simulink model "Example1_5"  (R2012a)
settings: Solver=ode45  StartTime=0.0  StopTime=T  MaxStep=MaxStep  RelTol=RelTol
values from neighbouring files (symbols this model uses):
  J = 20    [initialization_ex1_5.m]
  rule = 1    [initialization_ex1_5.m]
  T = 15    [initialization_ex1_5.m]
  x0 = [0; 0; pi/4; 2]    [initialization_ex1_5.m]
libraries: simulink x3
settings Model: Creator=pablonanez  LastModifiedBy=pablonanez
settings DataIOCC: LimitDataPoints=on  SaveFormat=Array  SignalLoggingSaveFormat=ModelDataLogs  ReturnWorkspaceOutputs=off
settings OptimizationCC: ExpressionDepthLimit=2147483647  LifeSpan=inf  SimCompilerOptimization=Off
settings DebuggingCC: UnderspecifiedInitializationDetection=Classic  MergeDetectMultiDrivingBlocksExec=none  SolverPrmCheckMsg=warning  FcnCallInpInsideContextMsg=Enable All  StateNameClashWarn=warning  SFUnexpectedBacktrackingDiag=warning  SFNoUnconditionalDefaultTransitionDiag=warning
settings HardwareCC: ProdBitPerPointer=32  ProdLargestAtomicFloat=None  ProdIntDivRoundTo=Undefined  ProdEndianess=Unspecified  ProdWordSize=32  ProdHWDeviceType=32-bit Generic
settings ModelReferenceCC: PropagateSignalLabelsOutOfModel=off
settings SFSimCC: SimUseLocalCustomCode=off  SimParseCustomCode=off
settings RTWCC: RTWUseLocalCustomCode=off  RTWCompilerOptimization=Off
settings GRTTargetCC: CodeReplacementLibrary=C89/C90 (ANSI)  GeneratePreprocessorConditionals=Disable all  CombineOutputUpdateFcns=off  CPPClassGenCompliant=off  GRTInterface=on

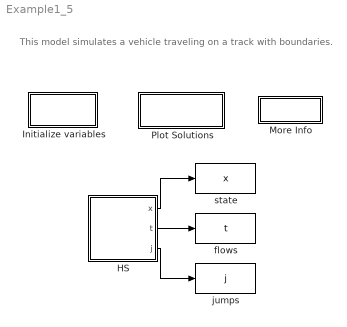
== system Example1_5 ==
  note: This model simulates a vehicle
      | traveling on a track with boundaries.
  HS : Subsystem  LoadFcn=set_param(gcb,'LinkStatus','none')
      settings: CopyFcn=|
      | set_param(gcb,'LinkStatus','none')
      | set_param(gcs, 'MaxStep', 'MaxStep', 'RelTol', 'RelTol')
      mask Display:
      | image(imread('Hcal.jpg'))
      | %plot([5 20 20 5 5],[5 5 20 20 5])
      | %text(8,13,'HyEq_mdl')
      | port_label('output', 1, 'x')
      | port_label('output', 2, 't')
      | port_label('output', 3, 'j')
  Initialize variables : Subsystem  Priority=-10
      settings: OpenFcn=initialization_ex1_5
      mask Display: disp('Double Click\n to Initialize')
  More Info : Subsystem
      settings: OpenFcn=web( 'Example_1_5.html')
      mask Display: disp('More Info')
  Plot Solutions : Subsystem
      settings: OpenFcn=postprocessing_ex1_5
      mask Display: disp('Double Click to\n Plot Solutions')
  flows : ToWorkspace  VariableName=t  SampleTime=-1
  jumps : ToWorkspace  VariableName=j  SampleTime=-1
  state : ToWorkspace  VariableName=x  SampleTime=-1
  wires:
  HS/2(t) -> flows/1
  HS/1(x) -> state/1
  HS/3(j) -> jumps/1

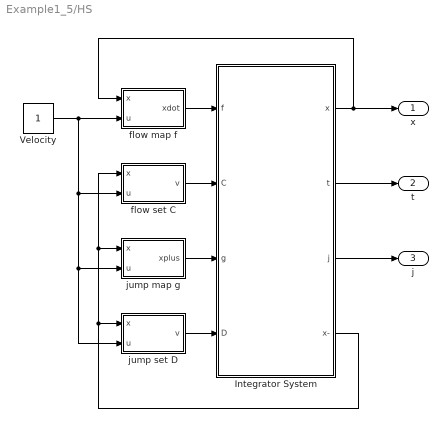
== system Example1_5/HS ==
  Integrator System : Subsystem  Priority=2  mask(Hybrid Integrator){T=T, J=J, x0=x0}
      mask prompts: T "Flow Horizon"; J "Jump Horizon"; x0 "Initial Condition"
      mask help:
      | This block integrates the state of the hybrid system defined by the flow map f (first input), the flow set C (second input), the jump map g (third input) and the jump set D (fourth input).
      | Starting from the initial condition x0 (last mask parameter), the system's state x evolves continuously within the set C, according to f(x,u), but is also subject to jumps within D, according to g(x,u).
      | The block also stops the simulation when the time t is greater than the flow horizon T (first mask parameter), or when the number of jumps j is greater than the jump horizon J (second mask parameter).
      | The outputs of the blocks are respectively x(t), t, j, x(t-).
      mask Help:
      | This block integrates the state of the hybrid system defined by the flow map f (first input), the flow set C (second input), the jump map g (third input) and the jump set D (fourth input).
      | <br>
      | Starting from the initial condition x0 (last mask parameter), the system's state x evolves continuously within the set C, according to f(x,u), but is also subject to jumps within D, according to g(x,u).
      | <br>
      | The block also stops the simulation when the time t is greater than the flow horizon T (first mask parameter), or when the number of jumps j is greater than the jump horizon J (second mask parameter).
      | <br>
      | The outputs of the blocks are respectively x(t), t, j, x(t-).
      | <br>
      | You can right click on the block and "Look under mask" to see what's inside the block.
      | Finally, refer to the manual (HybridSimulator_vXX.pdf) for more detailed information on how this hybrid simulator works.
  Velocity : Constant
  flow map f : MATLAB Function  TreatAsAtomicUnit=on
      settings: PermitHierarchicalResolution=ParametersOnly
  flow set C : MATLAB Function  TreatAsAtomicUnit=on
      settings: PermitHierarchicalResolution=ParametersOnly
  jump map g : MATLAB Function  Priority=2  TreatAsAtomicUnit=on
      settings: PermitHierarchicalResolution=ParametersOnly
  jump set D : MATLAB Function  TreatAsAtomicUnit=on
      settings: PermitHierarchicalResolution=ParametersOnly
  x : Outport
  t : Outport  Port=2
  j : Outport  Port=3
  wires:
  flow map f/1(xdot) -> Integrator System/1(f)
  Integrator System/4(x-) -> jump map g/1(x), flow set C/1(x), jump set D/1(x)
  Integrator System/1(x) -> flow map f/1(x), x/1
  flow set C/1(v) -> Integrator System/2(C)
  Integrator System/2(t) -> t/1
  Integrator System/3(j) -> j/1
  Velocity/1 -> flow map f/2(u), flow set C/2(u), jump map g/2(u), jump set D/2(u)
  jump set D/1(v) -> Integrator System/4(D)
  jump map g/1(xplus) -> Integrator System/3(g)

== system Example1_5/Initialize variables ==

== system Example1_5/More Info ==

== system Example1_5/Plot Solutions ==

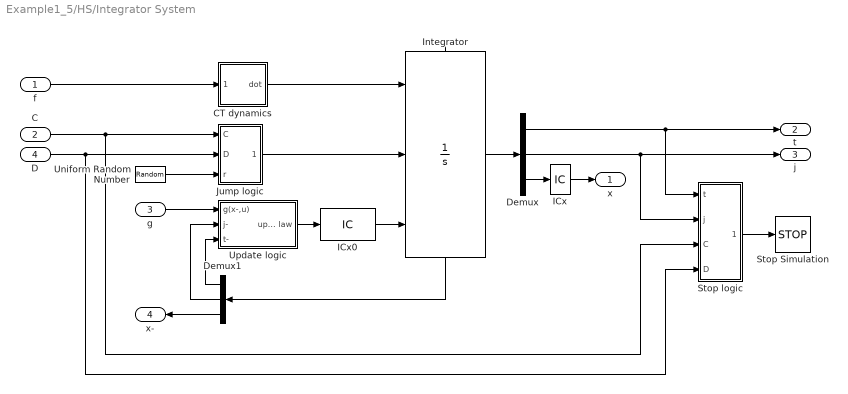
== system Example1_5/HS/Integrator System ==
  f : Inport
  C : Inport  Port=2
  g : Inport  Port=3
  D : Inport  Port=4
  CT dynamics : Subsystem
  Demux : Demux  Outputs=[1 1 -1]
  Demux1 : Demux  Outputs=[1 1 -1]
  ICx : InitialCondition  Value=x0
  ICx0 : InitialCondition  Value=[0; 0; x0(:)]
  Integrator : Integrator  ExternalReset=level hold  InitialConditionSource=external  ShowStatePort=on  ZeroCross=off
  Jump logic : Subsystem
  Stop Simulation : Stop
  Stop logic : Subsystem
  Uniform Random Number : UniformRandomNumber  Minimum=0  Seed=abs(floor(100*rand))  SampleTime=0
  Update logic : Subsystem
  x : Outport
  t : Outport  Port=2
  j : Outport  Port=3
  x- : Outport  Port=4
  wires:
  Demux1/2 -> Update logic/2(j-)
  Demux1/1 -> Update logic/3(t-)
  g/1 -> Update logic/1(g(x-,u))
  Uniform Random Number/1 -> Jump logic/3(r)
  Jump logic/1(jump) -> Integrator/2
  Demux1/3 -> x-/1
  f/1 -> CT dynamics/1(f(x,u))
  D/1 -> Jump logic/2(D), Stop logic/4(D)
  C/1 -> Jump logic/1(C), Stop logic/3(C)
  Integrator/1 -> Demux/1
  Stop logic/1(stop) -> Stop Simulation/1
  CT dynamics/1(dot) -> Integrator/1
  Update logic/1(update law) -> ICx0/1
  Demux/1 -> Stop logic/1(t), t/1
  Demux/2 -> Stop logic/2(j), j/1
  Integrator/State -> Demux1/1
  Demux/3 -> ICx/1
  ICx/1 -> x/1
  ICx0/1 -> Integrator/3

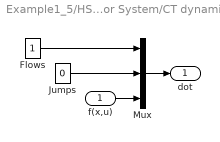
== system Example1_5/HS/Integrator System/CT dynamics ==
  f(x,u) : Inport
  Flows : Constant
  Jumps : Constant  Value=0
  Mux : Mux  Inputs=[1 1 -1]
  dot : Outport
  wires:
  f(x,u)/1 -> Mux/3
  Mux/1 -> dot/1
  Flows/1 -> Mux/1
  Jumps/1 -> Mux/2

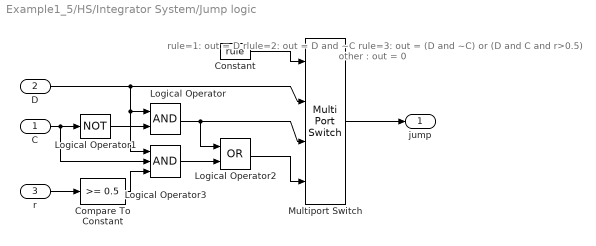
== system Example1_5/HS/Integrator System/Jump logic ==
  note: rule=1:  out = D
      | rlule=2: out = D and ~C
      | rule=3:  out = (D and ~C)  or (D and C and r>0.5)
      | other :  out = 0
  C : Inport
  D : Inport  Port=2
  r : Inport  Port=3
  Compare To Constant : simulink/Logic and Bit Operations/Compare To Constant  relop=>=  const=0.5  OutDataTypeStr=uint8
  Constant : Constant  Value=rule
  Logical Operator : Logic  AllPortsSameDT=off  OutDataTypeStr=boolean
  Logical Operator1 : Logic  Operator=NOT  Inputs=1  AllPortsSameDT=off  OutDataTypeStr=boolean
  Logical Operator2 : Logic  Operator=OR  AllPortsSameDT=off  OutDataTypeStr=boolean
  Logical Operator3 : Logic  Inputs=3  AllPortsSameDT=off  OutDataTypeStr=boolean
  Multiport Switch : MultiPortSwitch
  jump : Outport
  wires:
  Logical Operator3/1 -> Logical Operator2/2
  Compare To Constant/1 -> Logical Operator3/3
  Multiport Switch/1 -> jump/1
  Logical Operator2/1 -> Multiport Switch/4
  Logical Operator/1 -> Logical Operator2/1, Multiport Switch/3
  Logical Operator1/1 -> Logical Operator/2
  C/1 -> Logical Operator1/1, Logical Operator3/2
  r/1 -> Compare To Constant/1
  D/1 -> Multiport Switch/2, Logical Operator/1, Logical Operator3/1
  Constant/1 -> Multiport Switch/1

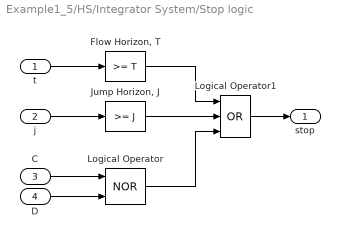
== system Example1_5/HS/Integrator System/Stop logic ==
  t : Inport
  j : Inport  Port=2
  C : Inport  Port=3
  D : Inport  Port=4
  "Flow Horizon, T" : simulink/Logic and Bit Operations/Compare To Constant  relop=>=  const=T  OutDataTypeStr=uint8  ZeroCross=off
  "Jump Horizon, J" : simulink/Logic and Bit Operations/Compare To Constant  relop=>=  const=J  OutDataTypeStr=uint8  ZeroCross=off
  Logical Operator : Logic  Operator=NOR  AllPortsSameDT=off  OutDataTypeStr=boolean
  Logical Operator1 : Logic  Operator=OR  Inputs=3  AllPortsSameDT=off  OutDataTypeStr=boolean
  stop : Outport
  wires:
  Logical Operator1/1 -> stop/1
  C/1 -> Logical Operator/1
  j/1 -> "Jump Horizon, J"/1
  t/1 -> "Flow Horizon, T"/1
  D/1 -> Logical Operator/2
  Logical Operator/1 -> Logical Operator1/3
  "Jump Horizon, J"/1 -> Logical Operator1/2
  "Flow Horizon, T"/1 -> Logical Operator1/1

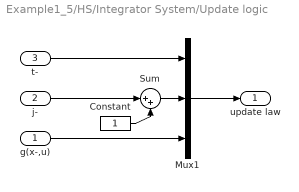
== system Example1_5/HS/Integrator System/Update logic ==
  g(x-,u) : Inport
  j- : Inport  Port=2
  t- : Inport  Port=3
  Constant : Constant
  Mux1 : Mux  Inputs=[1 1 -1]
  Sum : Sum  Inputs=|++
  update law : Outport
  wires:
  Constant/1 -> Sum/2
  t-/1 -> Mux1/1
  g(x-,u)/1 -> Mux1/3
  j-/1 -> Sum/1
  Mux1/1 -> update law/1
  Sum/1 -> Mux1/2

== matlab function Example1_5/HS/jump set D ==
  data: x input; v output; u input
function v  = D(x, u) 

%%%%%%%%%%%%%%%%%%%%%%%%%%%%%%%%%%%%%%%%%%%%%%%%%%%%%%%%%%%%%%%%%%%%%%%%%%%
% Matlab Function  Author: Ricardo Sanfelice
%
% Project: Simulation of a hybrid system (Vehicle Traveling on a Track)
%
% Name: D.m
%
% Description: Jump set
%
% Version: 1.0
% Required files: - 
%%%%%%%%%%%%%%%%%%%%%%%%%%%%%%%%%%%%%%%%%%%%%%%%%%%%%%%%%%%%%%%%%%%%%%%%%%%

xtemp = zeros(4,1);
xtemp = x;
x = xtemp;

% state
xi1 = x(1);      %x-position
xi2 = x(2);      %y-position
xi3 = x(3);      %orientation angle
q = x(4);  

% q = 1 --> going left
% q = 2 --> going right

 if ((xi1 >= 1) && (q == 2)) || ((xi1 <= -1) && (q == 1))  % jump condition
     v = 1;  % report jump
 else 
     v = 0; % do not report jump
 end

== matlab function Example1_5/HS/flow map f ==
  data: x input; xdot output; u input
function xdot = f(x, u)

%%%%%%%%%%%%%%%%%%%%%%%%%%%%%%%%%%%%%%%%%%%%%%%%%%%%%%%%%%%%%%%%%%%%%%%%%%%
% Matlab Function  Author: Ricardo Sanfelice
%
% Project: Simulation of a hybrid system (Vehicle Traveling on a Track)
%
% Name: f.m
%
% Description: Flow map
%
% Version: 1.0
% Required files: - 
%%%%%%%%%%%%%%%%%%%%%%%%%%%%%%%%%%%%%%%%%%%%%%%%%%%%%%%%%%%%%%%%%%%%%%%%%%%

xtemp = zeros(4,1);
xtemp = x;
x = xtemp;

% state
xi1 = x(1);      %x-position
xi2 = x(2);      %y-position
xi3 = x(3);      %orientation angle
q = x(4);       

% q = 1 --> going left
% q = 2 --> going right

if q == 1
    r = 3*pi/4;
elseif q == 2
    r = pi/4;
else
    r = 0;
end

% flow map: xidot=f(xi,u);
xi1dot = u*cos(xi3);  %tangential velocity in x-direction
xi2dot = u*sin(xi3);  %tangential velocity in y-direction
xi3dot = -xi3 + r;      %angular velocity
qdot = 0;

xdot = [xi1dot;xi2dot;xi3dot;qdot];

== matlab function Example1_5/HS/flow set C ==
  data: x input; v output; u input
function v  = C(x, u) 

%%%%%%%%%%%%%%%%%%%%%%%%%%%%%%%%%%%%%%%%%%%%%%%%%%%%%%%%%%%%%%%%%%%%%%%%%%%
% Matlab Function  Author: Ricardo Sanfelice
%
% Project: Simulation of a hybrid system (Vehicle Traveling on a Track)
%
% Name: C.m
%
% Description: Flow set
%
% Version: 1.0
% Required files: - 
%%%%%%%%%%%%%%%%%%%%%%%%%%%%%%%%%%%%%%%%%%%%%%%%%%%%%%%%%%%%%%%%%%%%%%%%%%%

xtemp = zeros(4,1);
xtemp = x;
x = xtemp;

% state
xi1 = x(1);      %x-position
xi2 = x(2);      %y-position
xi3 = x(3);      %orientation angle
q = x(4);  

% q = 1 --> going left
% q = 2 --> going right

if ((xi1 < 1) && (q == 2)) || ((xi1 > -1) && (q == 1))  % flow condition
    v = 1;  % report flow
else 
    v = 0;   % do not report flow
end

== matlab function Example1_5/HS/jump map g ==
  data: x input; xplus output; u input
function xplus = g(x, u)

%%%%%%%%%%%%%%%%%%%%%%%%%%%%%%%%%%%%%%%%%%%%%%%%%%%%%%%%%%%%%%%%%%%%%%%%%%%
% Matlab Function  Author: Ricardo Sanfelice
%
% Project: Simulation of a hybrid system (Vehicle Traveling on a Track)
%
% Name: g.m
%
% Description: Jump map
%
% Version: 1.0
% Required files: - 
%%%%%%%%%%%%%%%%%%%%%%%%%%%%%%%%%%%%%%%%%%%%%%%%%%%%%%%%%%%%%%%%%%%%%%%%%%%

xtemp = zeros(4,1);
xtemp = x;
x = xtemp;
% state
xi1 = x(1);      %x-position
xi2 = x(2);      %y-position
xi3 = x(3);      %orientation angle
q = x(4);  

% q = 1 --> going left
% q = 2 --> going right
xi1plus=xi1;
xi2plus=xi2;
xi3plus=xi3;
qplus=q;

% jump map
if ((xi1 >= 1) && (q == 2)) || ((xi1 <= -1) && (q == 1))
   qplus = 3-q;
else
    qplus = q;
end

xplus = [xi1plus;xi2plus;xi3plus;qplus];
